simulink subsystem "Gearbox"  (R2023a)
settings: Solver=VariableStepAuto  StartTime=0.0  StopTime=10.0  RelTol=1e-3
model mask{i=100, J_gear=2,4*10^-6, vis_friction_coef_gear=0.05}
  mask prompts: i "Gear ratio"; J_gear "Gear inertia"
values from neighbouring files (symbols this model uses):
  i_gear = 100    [constants.m]
  J_gear = 2.4 * 10^-6    (= 2.4e-06)    [constants.m]
  vis_friction_coef_gear = 0.05    [constants.m]
settings Model: Creator=ПК  LastModifiedBy=ycheb

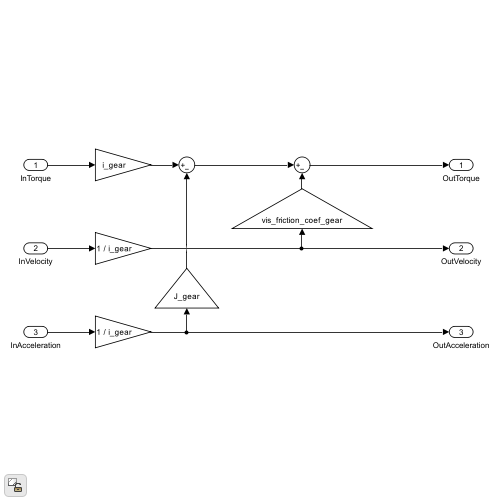
[thumbnail: Simulink's stored preview of the top-level diagram]
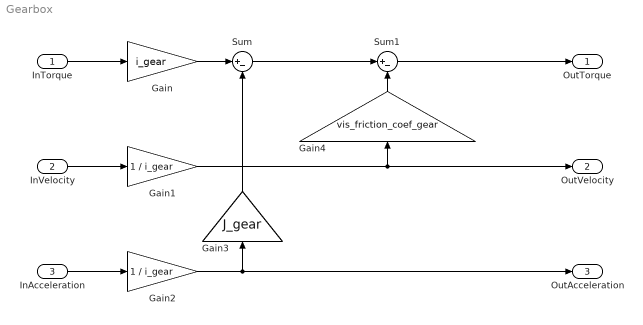
== system Gearbox ==
  InTorque : Inport
  InVelocity : Inport  Port=2
  InAcceleration : Inport  Port=3
  Gain : Gain  Gain=i_gear
  Gain1 : Gain  Gain=1 / i_gear
  Gain2 : Gain  Gain=1 / i_gear
  Gain3 : Gain  Gain=J_gear
  Gain4 : Gain  Gain=vis_friction_coef_gear
  Sum : Sum  Inputs=|+-
  Sum1 : Sum  Inputs=|+-
  OutTorque : Outport
  OutVelocity : Outport  Port=2
  OutAcceleration : Outport  Port=3
  wires:
  InTorque/1 -> Gain/1
  InVelocity/1 -> Gain1/1
  InAcceleration/1 -> Gain2/1
  Gain2/1 -> OutAcceleration/1, Gain3/1
  Gain1/1 -> OutVelocity/1, Gain4/1
  Gain/1 -> Sum/1
  Sum/1 -> Sum1/1
  Sum1/1 -> OutTorque/1
  Gain3/1 -> Sum/2
  Gain4/1 -> Sum1/2
